simulink model "inputGenerator"  (R2017a)
settings: Solver=VariableStepAuto  StartTime=0.0  StopTime=500  RelTol=1e-3
undefined symbols (not defined in the file or in its folder): denominator, numerator, timeDelay
settings Model: Creator=jpleitao  LastModifiedBy=jpleitao

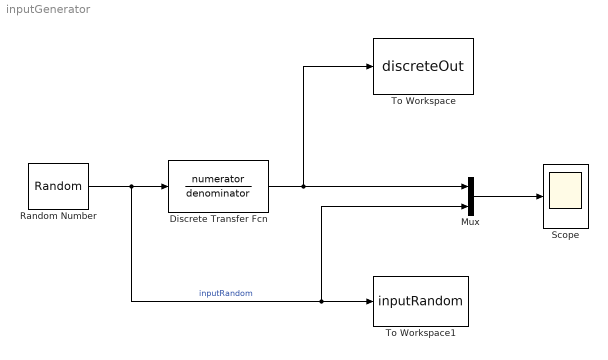
== system inputGenerator ==
  Discrete Transfer Fcn : DiscreteTransferFcn  Numerator=numerator  Denominator=denominator
  Mux : Mux  Inputs=2
  Random Number : RandomNumber  SampleTime=timeDelay
  Scope : Scope
  To Workspace : ToWorkspace  VariableName=discreteOut  SaveFormat=Timeseries  SampleTime=-1
  To Workspace1 : ToWorkspace  VariableName=inputRandom  SaveFormat=Timeseries  SampleTime=-1
  wires:
  Random Number/1 -> Mux/2, To Workspace1/1, Discrete Transfer Fcn/1  "inputRandom"
  Mux/1 -> Scope/1
  Discrete Transfer Fcn/1 -> To Workspace/1, Mux/1
